simulink model "watertank_FMU"  (Simulink 10.3)
settings: Solver=ode45  StartTime=0.0  StopTime=1000  RelTol=1e-3  EnableMultiTasking=on
settings Model: Creator=stefano  LastModifiedBy=filippo  MultithreadedSim=on
settings DataIOCC: LimitDataPoints=on  SignalLoggingSaveFormat=Dataset
settings OptimizationCC: ExpressionDepthLimit=128
settings DebuggingCC: UnderspecifiedInitializationDetection=Simplified  MergeDetectMultiDrivingBlocksExec=error  FcnCallInpInsideContextMsg=error  StateNameClashWarn=none
settings GRTTargetCC: CombineOutputUpdateFcns=on  GRTInterface=off

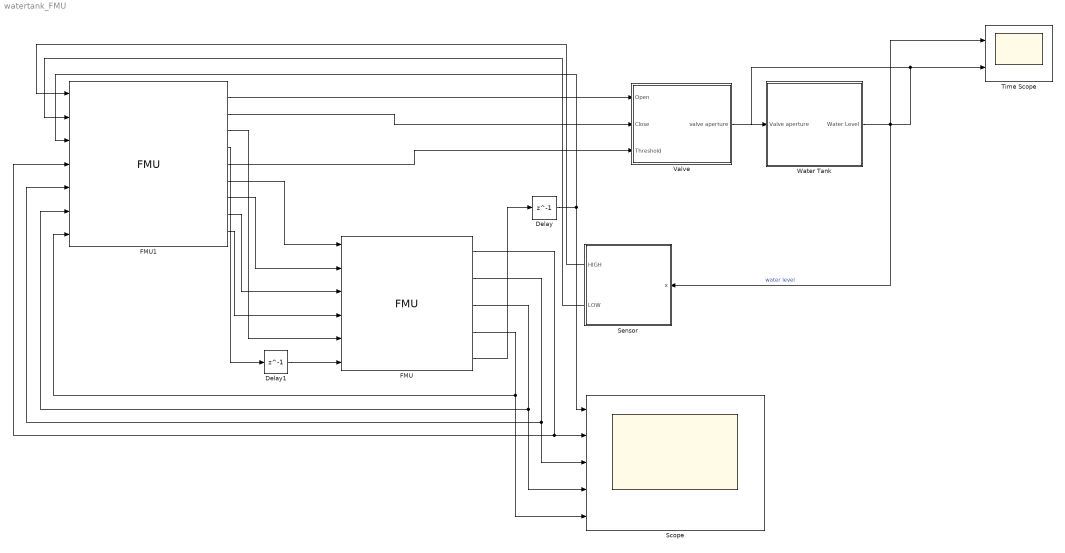
== system watertank_FMU ==
  Delay : Delay  DelayLength=1  InitialCondition=0
  Delay1 : Delay  DelayLength=1  InitialCondition=0
  FMU : FMU  FMUName=multiplicator_system.fmu  FMUDebugLoggingRedirect=Display  FMUDebugLoggingFilter=DataTag0  FMUMode=CoSimulation
      mask Type: multiplicator_system [Co-Simulation, v2.0]
      mask Display:
      | disp('multiplicator_system');
      | port_label('output',1,'Output_1');
      | port_label('output',2,'Output_2');
      | port_label('output',3,'Output_3');
      | port_label('output',4,'Output_4');
      | port_label('output',5,'Output_ready');
      | port_label('input',1,'Input_1');
      | port_label('input',2,'Input_2');
      | port_label('input',3,'Input_3');
      | port_label('input',4,'Input_4');
      | port_label('input',5,'Reset');
      | port_label('input',6,'Input_ready');
  FMU1 : FMU  FMUName=controller_system.fmu  FMUDebugLoggingRedirect=Display  FMUDebugLoggingFilter=DataTag1  FMUMode=CoSimulation
      mask Type: controller_system [Co-Simulation, v2.0]
      mask Display:
      | disp('controller_system');
      | port_label('output',1,'OPEN');
      | port_label('output',2,'CLOSE');
      | port_label('output',3,'reset');
      | port_label('output',4,'Input_ready');
      | port_label('output',5,'threshold');
      | port_label('output',6,'Input_1');
      | port_label('output',7,'Input_2');
      | port_label('output',8,'Input_3');
      | port_label('output',9,'Input_4');
      | port_label('input',1,'HIGH');
      | port_label('input',2,'LOW');
      | port_label('input',3,'Result_ready');
      | port_label('input',4,'Result_1');
      | port_label('input',5,'Result_2');
      | port_label('input',6,'Result_3');
      | port_label('input',7,'Result_4');
  Scope : Scope  NumInputPorts=5
  Sensor : Stateflow chart  TreatAsAtomicUnit=on
  Time Scope : Scope  NumInputPorts=2
  Valve : Subsystem
  Water Tank : Subsystem
  wires:
  Water Tank/1(Water Level) -> Sensor/1(x), Time Scope/1  "water level"
  Valve/1(valve aperture) -> Time Scope/2, Water Tank/1(Valve aperture)
  Sensor/1(HIGH) -> FMU1/1
  Sensor/2(LOW) -> FMU1/2
  FMU1/5 -> Valve/3(Threshold)
  FMU1/2 -> Valve/2(Close)
  FMU1/1 -> Valve/1(Open)
  FMU1/3 -> FMU/5
  FMU1/6 -> FMU/1
  FMU1/7 -> FMU/2
  FMU1/9 -> FMU/4
  FMU/5 -> Delay/1
  Delay/1 -> FMU1/3, Scope/1
  FMU/1 -> FMU1/4, Scope/2
  FMU/2 -> Scope/3, FMU1/5
  FMU/3 -> Scope/4, FMU1/6
  FMU/4 -> FMU1/7, Scope/5
  FMU1/8 -> FMU/3
  FMU1/4 -> Delay1/1
  Delay1/1 -> FMU/6

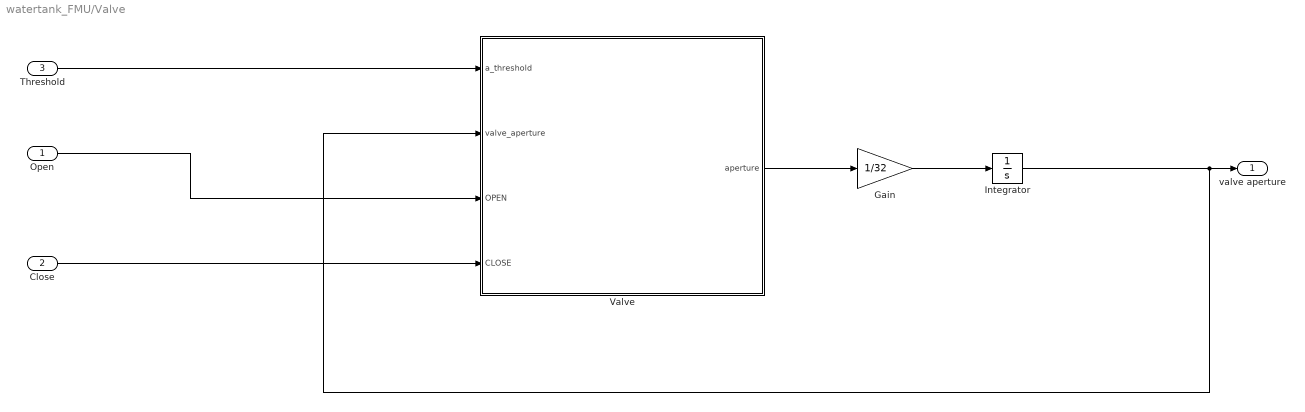
== system watertank_FMU/Valve ==
  Open : Inport
  Close : Inport  Port=2
  Threshold : Inport  Port=3  OutDataTypeStr=double
  Gain : Gain  Gain=1/32
  Integrator : Integrator  LimitOutput=on
  "Valve " : Stateflow chart  TreatAsAtomicUnit=on
  valve aperture : Outport  OutDataTypeStr=double
  wires:
  Threshold/1 -> "Valve "/1(a_threshold)
  "Valve "/1(aperture) -> Gain/1
  Gain/1 -> Integrator/1
  Integrator/1 -> valve aperture/1, "Valve "/2(valve_aperture)
  Open/1 -> "Valve "/3(OPEN)
  Close/1 -> "Valve "/4(CLOSE)

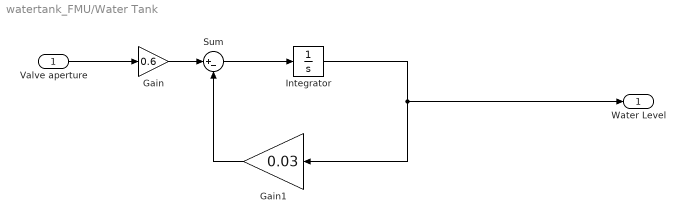
== system watertank_FMU/Water Tank ==
  Valve aperture : Inport
  Gain : Gain  Gain=0.6
  Gain1 : Gain  Gain=0.03
  Integrator : Integrator
  Sum : Sum  Inputs=|+-
  Water Level : Outport
  wires:
  Integrator/1 -> Gain1/1, Water Level/1
  Sum/1 -> Integrator/1
  Valve aperture/1 -> Gain/1
  Gain1/1 -> Sum/2
  Gain/1 -> Sum/1

== stateflow chart Valve/Valve  ==
  settings: updateMethod=DISCRETE  sampleTime=0.1
  state OPENING
    entry: aperture = 1
  state IDLE
    entry:  aperture = 0;
  state CLOSING
    entry: aperture = -1
  OPENING -> CLOSING [order 2] : [CLOSE == 1]
  IDLE -> OPENING [order 2] : [OPEN == 1]
  OPENING -> IDLE [order 1] : [valve_aperture>=a_threshold]
  CLOSING -> OPENING [order 2] : [OPEN == 1]
  (default) -> IDLE
  CLOSING -> IDLE [order 1] : [valve_aperture<=0]
  IDLE -> CLOSING [order 1] : [CLOSE==1]
  data: a_threshold input double; aperture output double; valve_aperture input double; OPEN input boolean; CLOSE input boolean

== stateflow chart Sensor ==
  settings: updateMethod=DISCRETE  sampleTime=0.1
  state EMPTY
    entry: LOW= false;
    entry: HIGH = false;
    entry: t=0;
    during: t= t+1;
  state FULL
    entry: HIGH= false;
    entry: LOW = false;
    entry: t=0;
    during: t= t+1;
  state SAFE
    entry: HIGH = false;
    entry: LOW = false;
  state EMPTY1
    entry: LOW = true;
  state FULL1
    entry: HIGH= true;
    ;
  EMPTY1 -> EMPTY
  EMPTY -> EMPTY1 [order 2] : [x<=Low & t >=5 ]
  FULL1 -> FULL
  FULL -> FULL1 [order 3] : [x>=High & t >=5]
  FULL -> EMPTY [order 2] : [x<=Low]
  SAFE -> EMPTY [order 2] : [x<=Low]
  EMPTY -> SAFE [order 1] : [x>Low]
  SAFE -> FULL [order 1] : [x>= High]
  FULL -> SAFE [order 1] : [x<= High]
  (default) -> SAFE
  data: Low constant single =5.5; x input double; High constant single =8; t local double; HIGH output boolean; LOW output boolean
